simulink model "HIL"  (R2023a)
settings: Solver=ode3  StartTime=0.0  StopTime=inf  FixedStep=0.01  RelTol=1e-3  EnableMultiTasking=on
undefined symbols (not defined in the file): gear_box_ratio, K
libraries: arduinolib x3, simulink_extras x2, arduinosensorlib x1
settings Model: SimulationMode=external  ExtModeTrigDuration=2  Creator=Shehab Abdo  LastModifiedBy=Shehab Abdo
settings SolverCC: AutoInsertRateTranBlk=on
settings OptimizationCC: EnhancedBackFolding=on  PassReuseOutputArgsAs=Individual arguments  ZeroExternalMemoryAtStartup=off  ZeroInternalMemoryAtStartup=off  MaxStackSize=64  OptimizeBlockOrder=speed  DifferentSizesBufferReuse=on  OptimizationCustomize=off  EfficientTunableParamExpr=on
settings DebuggingCC: MultiTaskRateTransMsg=warning  ParameterTunabilityLossMsg=error
settings HardwareCC: ProdBitPerInt=16  ProdBitPerPointer=16  ProdBitPerSizeT=16  ProdBitPerPtrDiffT=16  ProdLargestAtomicFloat=None  ProdWordSize=8  ProdHWDeviceType=Atmel->AVR
settings SFSimCC: MATLABDynamicMemAlloc=off
settings RTWCC: Description=Embedded Coder  SystemTargetFile=ert.tlc  HardwareBoard=Arduino Mega 2560  TemplateMakefile=ert_default_tmf  Toolchain=Arduino AVR  BuildConfiguration=Faster Runs
settings CodeAppCC: ForceParamTrailComments=on  IgnoreCustomStorageClasses=off  OperatorAnnotations=on  SimulinkDataObjDesc=on  SFDataObjDesc=on  InsertBlockDesc=on
settings ERTTargetCC: SupportContinuousTime=on  SupportVariableSizeSignals=on  ExtMode=on  ExtModeTransport=3  ExtModeStaticAlloc=on  ExtModeAutomaticAllocSize=off  ExtModeStaticAllocSize=2048  ExtModeMexFile=ext_xcp  ExtModeMexArgs=0 8 921600  ExtModeIntrfLevel=Level2 - Open

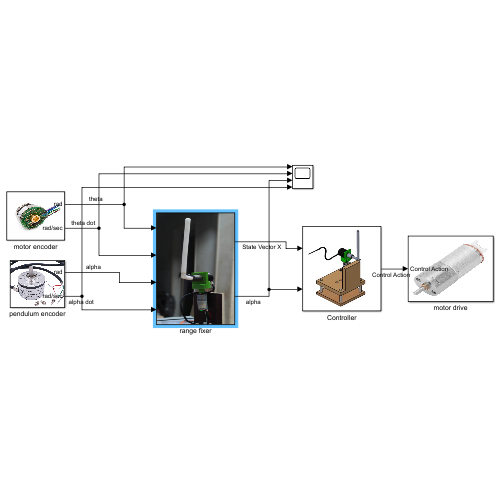
[thumbnail: Simulink's stored preview of the top-level diagram]
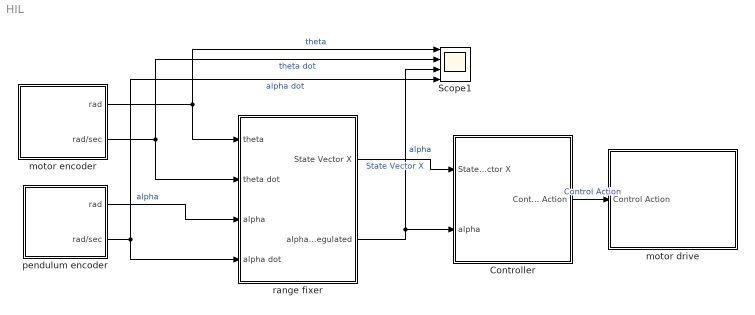
== system HIL ==
  Controller : Subsystem
      mask Display: image('D:\ASU\Hybird_Control\pandoll\img\setup.jpg'); % Use "Edit Image" on toolstrip to change.
  Scope1 : Scope  NumInputPorts=4
  motor drive : Subsystem
      mask Display: image('D:\ASU\Hybird_Control\pandoll\img\motor.jpg'); % Use "Edit Image" on toolstrip to change.
  motor encoder : Subsystem
      mask Display: image('D:\ASU\Hybird_Control\pandoll\img\motor encoder.jpg'); % Use "Edit Image" on toolstrip to change.
  pendulum encoder : Subsystem
      mask Display: image('D:\ASU\Hybird_Control\pandoll\img\encoder.jpg'); % Use "Edit Image" on toolstrip to change.
  range fixer : Subsystem
      mask Display: image('D:\ASU\Hybird_Control\pandoll\img\pendulum.png'); % Use "Edit Image" on toolstrip to change.
  wires:
  Controller/1("Control Action ") -> motor drive/1(Control Action)  "Control Action"
  range fixer/2("alpha_regulated ") -> Scope1/3, Controller/2(alpha)  "alpha"
  pendulum encoder/1(rad) -> range fixer/3(alpha)  "alpha"
  motor encoder/2(rad/sec) -> Scope1/2, range fixer/2(theta dot)  "theta dot"
  range fixer/1(State Vector X) -> Controller/1(State Vector X)  "State Vector X"
  motor encoder/1(rad) -> Scope1/1, range fixer/1(theta)  "theta"
  pendulum encoder/2(rad/sec) -> Scope1/4, range fixer/4(alpha dot)  "alpha dot"

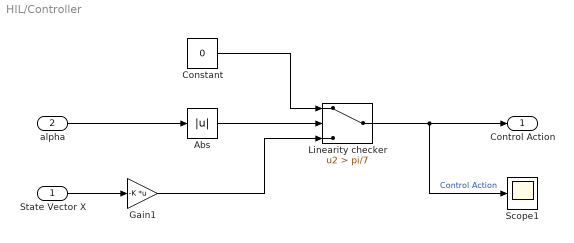
== system HIL/Controller ==
  State Vector X : Inport
  alpha : Inport  Port=2
  Abs : Abs  SaturateOnIntegerOverflow=off
  Constant : Constant  Value=0
  Gain1 : Gain  Gain=-K  Multiplication=Matrix(K*u)
  Linearity checker : Switch  Criteria=u2 > Threshold  Threshold=pi/7  SaturateOnIntegerOverflow=off  InputSameDT=off
  Scope1 : Scope
  "Control Action " : Outport
  wires:
  State Vector X/1 -> Gain1/1
  Constant/1 -> Linearity checker/1
  Linearity checker/1 -> "Control Action "/1, Scope1/1  "Control Action"
  Gain1/1 -> Linearity checker/3
  Abs/1 -> Linearity checker/2
  alpha/1 -> Abs/1

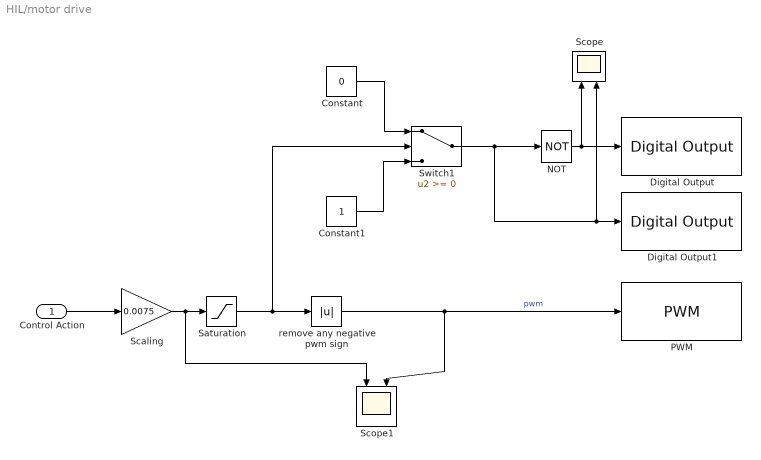
== system HIL/motor drive ==
  Control Action : Inport
  Constant : Constant  Value=0
  Constant1 : Constant
  Digital Output : arduinolib/Digital Output  pinNumber=7  Direction=output  blockPlatform=arduino
  Digital Output1 : arduinolib/Digital Output  pinNumber=8  Direction=output  blockPlatform=arduino
  NOT : Logic  Operator=NOT  IconShape=distinctive  AllPortsSameDT=off  OutDataTypeStr=boolean
  PWM : arduinolib/PWM  pinNumber=6  frequencyType=Default  desiredFrequency=490.2  achievableFrequency=490.2
  Saturation : Saturate  UpperLimit=255  LowerLimit=-255
  Scaling : Gain  Gain=0.0075
  Scope : Scope  NumInputPorts=2
  Scope1 : Scope  NumInputPorts=2
  Switch1 : Switch  SaturateOnIntegerOverflow=off  InputSameDT=off
  remove any negative pwm sign : Abs  SaturateOnIntegerOverflow=off
  wires:
  remove any negative pwm sign/1 -> PWM/1, Scope1/2  "pwm"
  Saturation/1 -> Switch1/2, remove any negative pwm sign/1
  Constant/1 -> Switch1/1
  Control Action/1 -> Scaling/1
  Scaling/1 -> Scope1/1, Saturation/1
  Constant1/1 -> Switch1/3
  Switch1/1 -> Digital Output1/1, Scope/2, NOT/1
  NOT/1 -> Digital Output/1, Scope/1

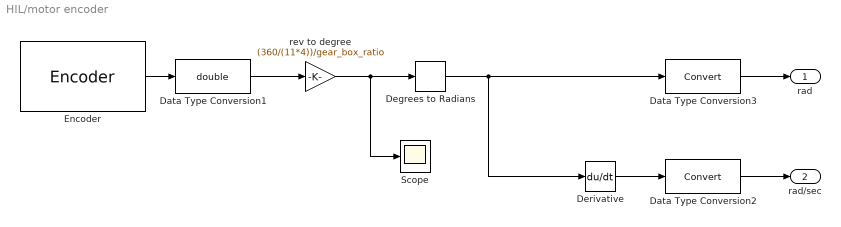
== system HIL/motor encoder ==
  Data Type Conversion1 : DataTypeConversion  OutDataTypeStr=double  SaturateOnIntegerOverflow=off  RndMeth=Floor
  Data Type Conversion2 : DataTypeConversion  SaturateOnIntegerOverflow=off  RndMeth=Floor
  Data Type Conversion3 : DataTypeConversion  SaturateOnIntegerOverflow=off  RndMeth=Floor
  Degrees to Radians : simulink_extras/Transformations/Degrees to Radians
  Derivative : Derivative
  Encoder : arduinosensorlib/Encoder  InputA=2  InputB=3  Mode=No reset  SampleTime=-1
  Scope : Scope
  rev to degree : Gain  Gain=(360/(11*4))/gear_box_ratio
  rad : Outport
  rad/sec : Outport  Port=2
  wires:
  Derivative/1 -> Data Type Conversion2/1
  rev to degree/1 -> Scope/1, Degrees to Radians/1
  Degrees to Radians/1 -> Derivative/1, Data Type Conversion3/1
  Data Type Conversion3/1 -> rad/1
  Data Type Conversion2/1 -> rad/sec/1
  Data Type Conversion1/1 -> rev to degree/1
  Encoder/1 -> Data Type Conversion1/1

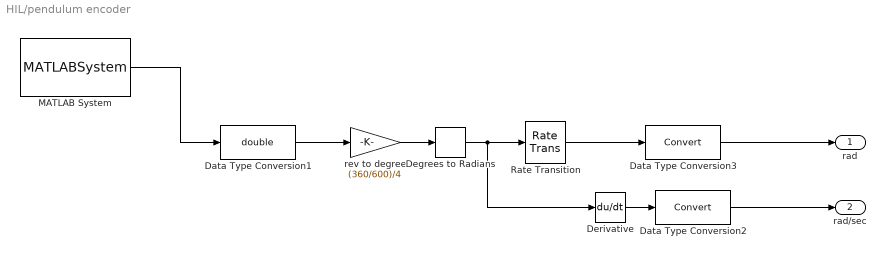
== system HIL/pendulum encoder ==
  Data Type Conversion1 : DataTypeConversion  OutDataTypeStr=double  SaturateOnIntegerOverflow=off  RndMeth=Floor
  Data Type Conversion2 : DataTypeConversion  SaturateOnIntegerOverflow=off  RndMeth=Floor
  Data Type Conversion3 : DataTypeConversion  SaturateOnIntegerOverflow=off  RndMeth=Floor
  Degrees to Radians : simulink_extras/Transformations/Degrees to Radians
  Derivative : Derivative
  MATLAB System : MATLABSystem  System=Encoder_arduino  Encoder=0  PinA=18  PinB=19  SampleTime=0.01
      mask Type: Encoder_arduino
      mask Display:
      | disp('Encoder');
      | port_label('output',1,'y');
  Rate Transition : RateTransition
  rev to degree : Gain  Gain=(360/600)/4
  rad : Outport
  rad/sec : Outport  Port=2
  wires:
  Data Type Conversion3/1 -> rad/1
  Data Type Conversion2/1 -> rad/sec/1
  Data Type Conversion1/1 -> rev to degree/1
  rev to degree/1 -> Degrees to Radians/1
  Derivative/1 -> Data Type Conversion2/1
  Degrees to Radians/1 -> Derivative/1, Rate Transition/1
  MATLAB System/1 -> Data Type Conversion1/1
  Rate Transition/1 -> Data Type Conversion3/1

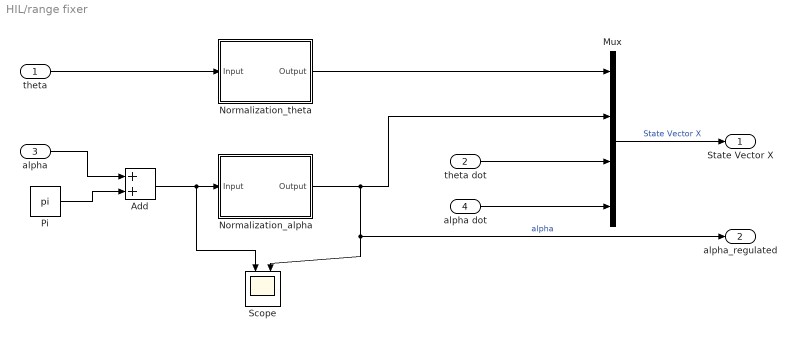
== system HIL/range fixer ==
  theta : Inport
  theta dot : Inport  Port=2
  alpha : Inport  Port=3
  alpha dot : Inport  Port=4
  Add : Sum
  Mux : Mux
  Normalization_alpha : Subsystem
  Normalization_theta : Subsystem
  Pi : Constant  Value=pi  OutDataTypeStr=Inherit: Inherit via back propagation
  Scope : Scope  NumInputPorts=2
  State Vector X : Outport
  "alpha_regulated " : Outport  Port=2
  wires:
  theta/1 -> Normalization_theta/1(Input)
  Mux/1 -> State Vector X/1  "State Vector X"
  Normalization_theta/1(Output) -> Mux/1
  alpha dot/1 -> Mux/4
  Pi/1 -> Add/2
  Add/1 -> Normalization_alpha/1(Input), Scope/1
  Normalization_alpha/1(Output) -> Mux/2, "alpha_regulated "/1, Scope/2  "alpha"
  alpha/1 -> Add/1
  theta dot/1 -> Mux/3

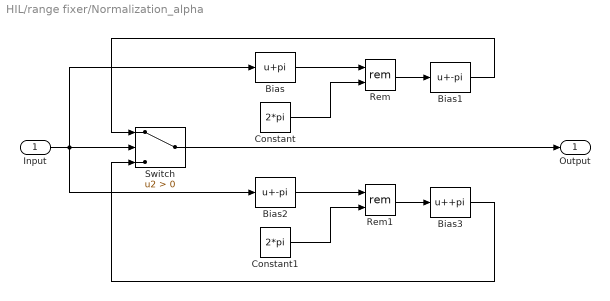
== system HIL/range fixer/Normalization_alpha ==
  Input : Inport
  Bias : Bias  Bias=pi  SaturateOnIntegerOverflow=off
  Bias1 : Bias  Bias=-pi  SaturateOnIntegerOverflow=off
  Bias2 : Bias  Bias=-pi  SaturateOnIntegerOverflow=off
  Bias3 : Bias  Bias=+pi  SaturateOnIntegerOverflow=off
  Constant : Constant  Value=2*pi
  Constant1 : Constant  Value=2*pi
  Rem : Math  Operator=rem  SignedPower=on
  Rem1 : Math  Operator=rem  SignedPower=on
  Switch : Switch  Criteria=u2 > Threshold  SaturateOnIntegerOverflow=off  InputSameDT=off
  Output : Outport
  wires:
  Constant/1 -> Rem/2
  Bias/1 -> Rem/1
  Input/1 -> Bias/1, Bias2/1, Switch/2
  Bias3/1 -> Switch/3
  Bias2/1 -> Rem1/1
  Rem1/1 -> Bias3/1
  Constant1/1 -> Rem1/2
  Switch/1 -> Output/1
  Rem/1 -> Bias1/1
  Bias1/1 -> Switch/1

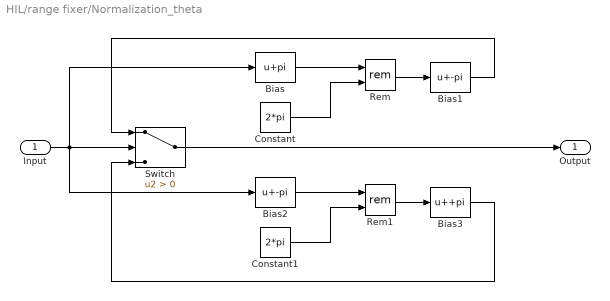
== system HIL/range fixer/Normalization_theta ==
  Input : Inport
  Bias : Bias  Bias=pi  SaturateOnIntegerOverflow=off
  Bias1 : Bias  Bias=-pi  SaturateOnIntegerOverflow=off
  Bias2 : Bias  Bias=-pi  SaturateOnIntegerOverflow=off
  Bias3 : Bias  Bias=+pi  SaturateOnIntegerOverflow=off
  Constant : Constant  Value=2*pi
  Constant1 : Constant  Value=2*pi
  Rem : Math  Operator=rem  SignedPower=on
  Rem1 : Math  Operator=rem  SignedPower=on
  Switch : Switch  Criteria=u2 > Threshold  SaturateOnIntegerOverflow=off  InputSameDT=off
  Output : Outport
  wires:
  Constant/1 -> Rem/2
  Bias/1 -> Rem/1
  Input/1 -> Bias/1, Bias2/1, Switch/2
  Bias3/1 -> Switch/3
  Bias2/1 -> Rem1/1
  Rem1/1 -> Bias3/1
  Constant1/1 -> Rem1/2
  Switch/1 -> Output/1
  Rem/1 -> Bias1/1
  Bias1/1 -> Switch/1
